simulink model "ReadWrite_Demo"  (Simulink 8.1)
settings: Solver=FixedStepDiscrete  StartTime=0.0  StopTime=10.0  FixedStep=0.1  RelTol=1e-3
undefined symbols (not defined in the file or in its folder): A14, A7, B, B13, D, L3, PD3, PD7, R10, R4
libraries: rappid_564xl_ec_toolbox x7, simulink x2
settings Model: Creator=B37386  LastModifiedBy=evarshavskaya
settings DataIOCC: ExternalInput=off  InitialState=off  SaveOutput=off  SignalLogging=off  SaveTime=off
settings OptimizationCC: InlineParams=on  OptimizeModelRefInitCode=on  LifeSpan=1
settings DebuggingCC: InheritedTsInSrcMsg=none  SingleTaskRateTransMsg=error  UnconnectedInputMsg=error  UnconnectedOutputMsg=error  UnconnectedLineMsg=error  UnknownTsInhSupMsg=error  StrictBusMsg=Warning
settings HardwareCC: ProdLargestAtomicInteger=Long  ProdLargestAtomicFloat=Double  ProdIntDivRoundTo=Zero  ProdEndianess=BigEndian  ProdHWDeviceType=Freescale->32-bit PowerPC
settings RTWCC: SystemTargetFile=rappid564xl.tlc  MakeCommand=rappid_564xl_make_rtw  TemplateMakefile=rappid_564xl_default_tmf  PostCodeGenCommand=rappid_analyzegencode(buildInfo)  Description=RAppID Toolbox MPC564xL Code Generation Target (rappid)  ProcessScript=rappid564xl_make_rtw_hook
settings CodeAppCC: IgnoreCustomStorageClasses=off  CustomSymbolStrType=$N$R$M  InternalIdentifier=Classic
settings STFCustomTargetCC: CodeReplacementLibrary=ANSI_C  CombineOutputUpdateFcns=on  SuppressErrorStatus=on  ERTCustomFileBanners=on  SupportContinuousTime=off  SupportNonInlinedSFcns=off  MATLABClassNameForMDSCustomization=Simulink.SoftwareTarget.ERTCustomization  GRTInterface=off  SystemTargetFile=rappid564xl.tlc
settings ERTTargetCC: CodeReplacementLibrary=ANSI_C  MultiwordLength=2048  ParMdlRefBuildCompliant=off  CompOptLevelCompliant=off  ConcurrentExecutionCompliant=off  SuppressErrorStatus=on  ERTFirstTimeCompliant=off  ModelStepFunctionPrototypeControlCompliant=off  CPPClassGenCompliant=off  InlinedParameterPlacement=NonHierarchical  ERTCustomFileTemplate=example_file_process.tlc  ConvertIfToSwitch=off  SuppressUnreachableDefaultCases=off

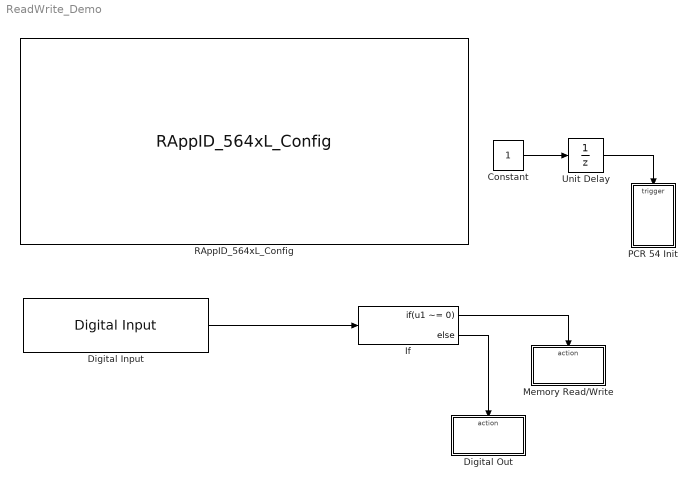
== system ReadWrite_Demo ==
  Constant : Constant  OutDataTypeStr=boolean
  Digital Input : rappid_564xl_ec_toolbox/MPC564xL/General Purpose Blocks/Digital Input  gpio_outputs="51  : PD3  : [ 128 ] : [ A7 ]"  pinNum=[ 128 ]  pcrNum=51
  Digital Out : Subsystem  TreatAsAtomicUnit=on
  If : If  IfExpression=u1 ~= 0
  Memory Read/Write : Subsystem  TreatAsAtomicUnit=on
  PCR 54 Init : Subsystem
  RAppID_564xL_Config : rappid_564xl_ec_toolbox/MPC564xL/RAppID_564xL_Config  SystemClock=120  XTAL=40  MC_clock_60=12  MC_clock_80=16  MC_clock_120=10  SWG_clock_60=20  SWG_clock_80=13.334  SWG_clock_120=20  Compiler=CodeWarrior  MemTarget=RAM  Part=MPC5643L  Package=144 LQFP  global_int_priority=10  base_tick_priority=11  sys_task_supress=off  exception_handlers=off  stored_mdl_name=ReadWrite_Demo  freemaster_interface=Oops  freemaster_rx_pin="LINFlex_0 Rx Pin 116 : \"PB[3]\""  freemaster_tx_pin="LINFlex_0 Tx Pin 114 : \"PB[2]\""  freemaster_interface_1=Serial 0  freemaster_enable=on  freemaster_rate=57600  freemaster_tx0_pin=18 : B[2] : 114 : A14  freemaster_rx0_pin=19 : B[3] : 116 : B13  freemaster_tx1_pin=57 : D[9] : 26 : L3  freemaster_rx1_pin=29 : B[13] : 60 : R10  freemaster_can_channel=1CH  freemater_can_speed=500K  freemaster_can_msgig=0x7AA  ccp_interface=None  ccp_enable=off  ccp_can_channel=CH1 (MB 0 - 1)  ccp_can_speed=500K  ccp_can_cro_id=256  ccp_can_dto_id=257  ccp_dev_id=RappID  ccp_dev_addr=0  ccp_odt=3  ccp_daq=3  pil_enable=off  pil_bam=off  comport=1  pil_rate=115200  bam_password_def=on  bam_password=0xFEEDFACECAFEBEEF  bam_sa_cs=off  bam_start_address=0x0  bam_code_size=0x7000  cons_dspi=on  cons_can=on  cons_adc=on  cons_pwm=on  cons_ctu=on  cons_swg=on  cons_eTimer=on  cons_fm=on
  Unit Delay : UnitDelay  SampleTime=-1
  wires:
  Digital Input/1 -> If/1
  If/1 -> Memory Read/Write/Action
  If/2 -> Digital Out/Action
  Constant/1 -> Unit Delay/1
  Unit Delay/1 -> PCR 54 Init/Trigger

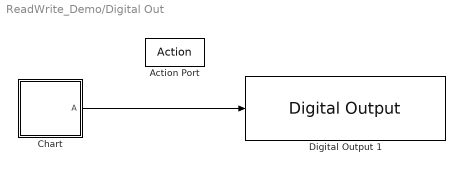
== system ReadWrite_Demo/Digital Out ==
  Action Port : ActionPort  ActionType=else
  Chart : Stateflow chart  TreatAsAtomicUnit=on
  Digital Output 1 : rappid_564xl_ec_toolbox/MPC564xL/General Purpose Blocks/Digital Output   gpio_outputs="55  : PD7  : [ 37 ] : [ R4 ]"  pinNum=[ 37 ]  pcrNum=55
  wires:
  Chart/1(A) -> Digital Output 1/1

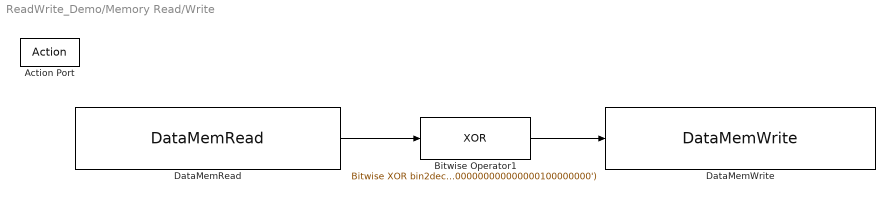
== system ReadWrite_Demo/Memory Read/Write ==
  Action Port : ActionPort  ActionType=then
  Bitwise Operator1 : simulink/Logic and Bit Operations/Bitwise Operator  logicop=XOR  UseBitMask=on  BitMask=bin2dec('00000000000000000000000100000000')  BitMaskRealWorld=Stored Integer
  DataMemRead : rappid_564xl_ec_toolbox/MPC564xL/Utility Blocks/DataMemRead  base_address=C3F90000  offset=634  ba=3287875584  off=1588
  DataMemWrite : rappid_564xl_ec_toolbox/MPC564xL/Utility Blocks/DataMemWrite  base_address=C3F90000  offset=634  ba=3287875584  off=1588
  wires:
  Bitwise Operator1/1 -> DataMemWrite/1
  DataMemRead/1 -> Bitwise Operator1/1

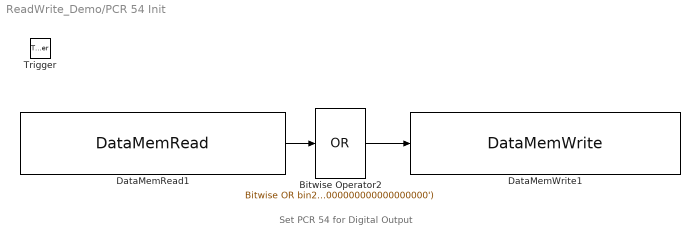
== system ReadWrite_Demo/PCR 54 Init ==
  note: Set PCR 54 for Digital Output
  Trigger : TriggerPort
  Bitwise Operator2 : simulink/Logic and Bit Operations/Bitwise Operator  logicop=OR  UseBitMask=on  BitMask=bin2dec('00000011000000000000000000000000')  BitMaskRealWorld=Stored Integer
  DataMemRead1 : rappid_564xl_ec_toolbox/MPC564xL/Utility Blocks/DataMemRead  base_address=C3F90000  offset=AC  ba=3287875584  off=172
  DataMemWrite1 : rappid_564xl_ec_toolbox/MPC564xL/Utility Blocks/DataMemWrite  base_address=C3F90000  offset=AC  ba=3287875584  off=172
  wires:
  DataMemRead1/1 -> Bitwise Operator2/1
  Bitwise Operator2/1 -> DataMemWrite1/1

== stateflow chart Digital Out/Chart ==
  state A [parallel]
    settings: executionOrder=1
    state A
    state A1
    (default) -> A.A
    A.A -> A1
    A1 -> A.A
  data: A output boolean [0..1]
